simulink model "invertedpendulumLQR"  (R2025a)
settings: Solver=VariableStepAuto  StartTime=0.0  StopTime=22  RelTol=1e-3
values from neighbouring files (symbols this model uses):
  A = [0 1 0 0 ... (first row only)    [invertedpendulum.m]
  B = [0; 1/M; 0; -1/(M*L)]    [invertedpendulum.m]
  D = zeros(4,1)    [invertedpendulum.m]
  K = lqr(A, B, Q, R)    [invertedpendulum.m]
settings Model: Creator=zackk  LastModifiedBy=zackk
settings DataIOCC: ReturnWorkspaceOutputs=off

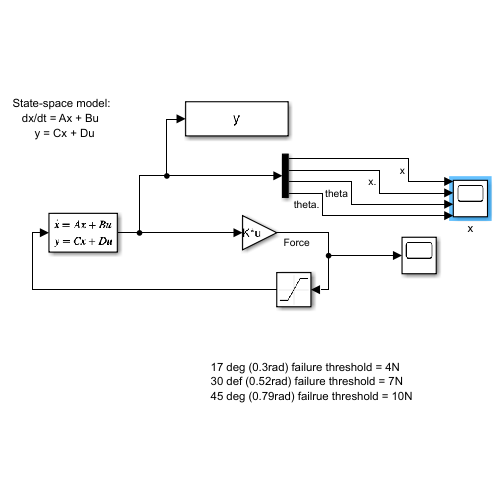
[thumbnail: Simulink's stored preview of the top-level diagram]
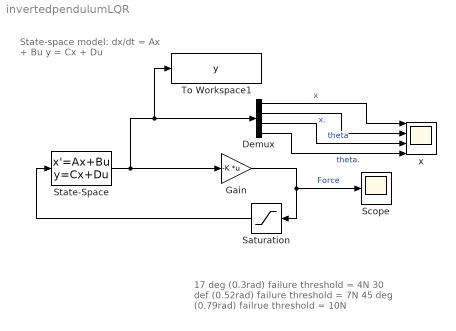
== system invertedpendulumLQR ==
  note: 17 deg (0.3rad) failure threshold = 4N
      | 30 def (0.52rad) failure threshold = 7N
      | 45 deg (0.79rad) failrue threshold = 10N
  note: State-space model:
      | dx/dt = Ax + Bu
      | y = Cx + Du
  Demux : Demux
  Gain : Gain  Gain=-K  Multiplication=Matrix(K*u)
  Saturation : Saturate  UpperLimit=6  LowerLimit=-6
  Scope : Scope
      settings: ActiveDisplayYMinimum=-8.0392516032503545E+30  ActiveDisplayYMaximum=7.2353264429253211E+31
  State-Space : StateSpace  A=A  B=B  C=eye(4)  D=D  InitialCondition=[0 ;0 ; 0.52; 0]
  To Workspace1 : ToWorkspace  VariableName=y  SampleTime=-1
      settings: Save2DSignal=2-D array (concatenate along first dimension)
  x : Scope  NumInputPorts=4
      settings: ActiveDisplayYMinimum=-9.811779347790705E+41  ActiveDisplayYMaximum=5.0927807090913666E+42
  wires:
  State-Space/1 -> To Workspace1/1, Demux/1, Gain/1
  Demux/1 -> x/1  "x"
  Demux/2 -> x/2  "x."
  Demux/3 -> x/3  "theta"
  Demux/4 -> x/4  "theta."
  Saturation/1 -> State-Space/1
  Gain/1 -> Scope/1, Saturation/1  "Force"
